simulink model "controllerComputedTorque"  (Simulink 8.0)
settings: Solver=FixedStepDiscrete  StartTime=0.0  StopTime=inf  FixedStep=1  RelTol=1e-3
InitFcn:
  | initSharedMem;
values from neighbouring files (symbols this model uses):
  k_pst = [ diag([k_pst_torso k_pst_arm k_pst_arm k_pst_leg k_pst_leg])    0*eye(25)   0*eye(25)]    [initCompleteForceControlSim.m]    (also in initPartialForceControl.m; initPartialForceControlSim.m)
  nj = 25    [initCompleteForceControlSim.m]    (also in initMonitor.m; initMonitorSim.m; initPartialForceControl.m; initPartialForceControlSim.m)
undefined symbols (not defined in the file or in its folder): DiscIntNeverNeededParam, k_com, k_pos
libraries: WBCLibrary x12, simulink x2, dspsigops x1
settings Model: Creator=daniele  LastModifiedBy=daniele
settings DebuggingCC: FcnCallInpInsideContextMsg=EnableAllAsWarning
settings GRTTargetCC: CombineOutputUpdateFcns=off  GRTInterface=on

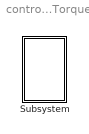
== system controllerComputedTorque ==
  Subsystem : Subsystem  mask{robotName='icub', Ts=0.01, localName='dynamicBalancing'}
      mask prompts: robotName "robot name"; localName "module name"

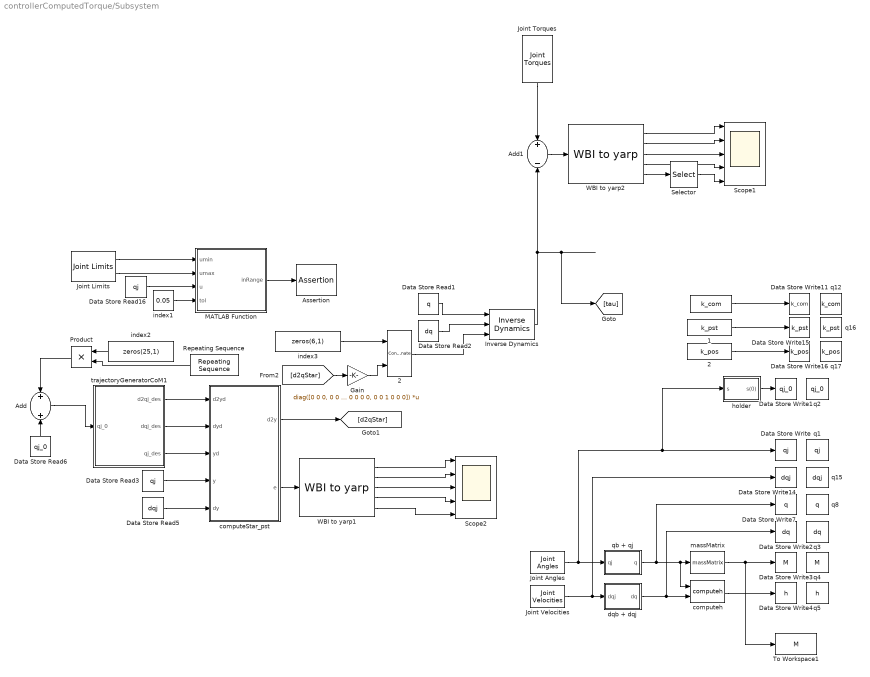
== system controllerComputedTorque/Subsystem ==
  "    " : Constant  Value=k_com
  "    1" : Constant  Value=k_pst
  "    2" : Constant  Value=k_pos
  " 2" : Concatenate  Mode=Multidimensional array
  Add : Sum  Inputs=+|+
  Add1 : Sum  Inputs=+|-
  Assertion : Assertion  Enabled=on
  Data Store Read1 : DataStoreRead  DataStoreName=q
  Data Store Read16 : DataStoreRead  DataStoreName=qj
  Data Store Read2 : DataStoreRead  DataStoreName=dq
  Data Store Read3 : DataStoreRead  DataStoreName=qj
  Data Store Read5 : DataStoreRead  DataStoreName=dqj
  Data Store Read6 : DataStoreRead  DataStoreName=qj_0
  Data Store Write : DataStoreWrite  Priority=-1  DataStoreName=qj
  Data Store Write1 : DataStoreWrite  Priority=-1  DataStoreName=qj_0
  Data Store Write11 : DataStoreWrite  Priority=-1  DataStoreName=k_com
  Data Store Write14 : DataStoreWrite  Priority=-1  DataStoreName=dqj
  Data Store Write15 : DataStoreWrite  Priority=-1  DataStoreName=k_pst
  Data Store Write16 : DataStoreWrite  Priority=-1  DataStoreName=k_pos
  Data Store Write2 : DataStoreWrite  Priority=-1  DataStoreName=dq
  Data Store Write3 : DataStoreWrite  Priority=-1  DataStoreName=M
  Data Store Write4 : DataStoreWrite  Priority=-1  DataStoreName=h
  Data Store Write7 : DataStoreWrite  Priority=-1  DataStoreName=q
  Gain : Gain  Gain=diag([0 0 0, 0 0 0 0 0, 0 0 0 0 0, 0 0 0 0 0 0, 0 0 1 0 0 0])  Multiplication=Matrix(K*u)
  Inverse Dynamics : WBCLibrary/wholeBodyModel/Dynamics/Inverse Dynamics  robotName=robotName  localName=localName
  Joint Angles : WBCLibrary/wholeBodyStates/Joint Angles  robotName=robotName  localName=localName
  Joint Limits : WBCLibrary/wholeBodyModel/Joint Limits  robotName=robotName  localName=localName
  Joint Torques : WBCLibrary/wholeBodyStates/Joint Torques  robotName=robotName  localName=localName
  Joint Velocities : WBCLibrary/wholeBodyStates/Joint Velocities  robotName=robotName  localName=localName
  MATLAB Function : MATLAB Function  TreatAsAtomicUnit=on
  Product : Product  RndMeth=Zero
  Repeating Sequence : simulink/Sources/Repeating Sequence  rep_seq_t=[0 1 2 3 4 ].*1000  rep_seq_y=[0 0 -0.1 -0.1 0]
  Scope1 : Scope  NumInputPorts=5
      settings: TimeRange=1400  YMin=-1~-0.5~-0.8~-0.2~-0.1  YMax=4~0.2~0.2~0.4~0.5
  Scope2 : Scope  NumInputPorts=5
      settings: TimeRange=1400  YMin=-0.5~-0.35~-0.6~-0.2~-0.75  YMax=3~0.1~0.1~0.3~0.75
  Selector : Selector  InputPortWidth=6  IndexOptions=Index vector (dialog)  Indices=[2 3]  OutputSizes=1
  To Workspace1 : ToWorkspace  VariableName=M  SampleTime=-1  SaveFormat=Structure
  WBI to yarp1 : WBCLibrary/Utilities/WBI to yarp
  WBI to yarp2 : WBCLibrary/Utilities/WBI to yarp
  computeStar_pst : Subsystem  mask{Kp=k_pst(1:25,1:25), Kd=k_pst(1:25,26:50), Ki=k_pst(1:25,51:75)}
  computeh : WBCLibrary/wholeBodyModel/Dynamics/computeh  val=7  robotname=robotName  localname=localName
  dqb + dqj : Subsystem
  holder : Subsystem
  index1 : Constant  Value=0.05  VectorParams1D=off
  index2 : Constant  Value=zeros(25,1)  VectorParams1D=off
  index3 : Constant  Value=zeros(6,1)  VectorParams1D=off
  massMatrix : WBCLibrary/wholeBodyModel/Dynamics/massMatrix  val=8  robotname=robotName  localname=localName
  q1 : DataStoreMemory  Priority=-1  DataStoreName=qj  ReadBeforeWriteMsg=warning  WriteAfterWriteMsg=warning  WriteAfterReadMsg=warning  InitialValue=zeros(nj,1)  VectorParams1D=off  OutDataTypeStr=double
  q12 : DataStoreMemory  Priority=-1  DataStoreName=k_com  ReadBeforeWriteMsg=warning  WriteAfterWriteMsg=warning  WriteAfterReadMsg=warning  InitialValue=k_com  VectorParams1D=off  OutDataTypeStr=double
  q15 : DataStoreMemory  Priority=-1  DataStoreName=dqj  ReadBeforeWriteMsg=warning  WriteAfterWriteMsg=warning  WriteAfterReadMsg=warning  InitialValue=zeros(nj,1)  VectorParams1D=off  OutDataTypeStr=double
  q16 : DataStoreMemory  Priority=-1  DataStoreName=k_pst  ReadBeforeWriteMsg=warning  WriteAfterWriteMsg=warning  WriteAfterReadMsg=warning  InitialValue=k_pst  VectorParams1D=off  OutDataTypeStr=double
  q17 : DataStoreMemory  Priority=-1  DataStoreName=k_pos  ReadBeforeWriteMsg=warning  WriteAfterWriteMsg=warning  WriteAfterReadMsg=warning  InitialValue=k_pos  VectorParams1D=off  OutDataTypeStr=double
  q2 : DataStoreMemory  Priority=-1  DataStoreName=qj_0  ReadBeforeWriteMsg=warning  WriteAfterWriteMsg=warning  WriteAfterReadMsg=warning  InitialValue=zeros(nj,1)  VectorParams1D=off  OutDataTypeStr=double
  q3 : DataStoreMemory  Priority=-1  DataStoreName=dq  ReadBeforeWriteMsg=warning  WriteAfterWriteMsg=warning  WriteAfterReadMsg=warning  InitialValue=zeros(nj+6,1)  VectorParams1D=off  OutDataTypeStr=double
  q4 : DataStoreMemory  Priority=-1  DataStoreName=M  ReadBeforeWriteMsg=warning  WriteAfterWriteMsg=warning  WriteAfterReadMsg=warning  InitialValue=zeros(nj+6,nj+6)  VectorParams1D=off  OutDataTypeStr=double
  q5 : DataStoreMemory  Priority=-1  DataStoreName=h  ReadBeforeWriteMsg=warning  WriteAfterWriteMsg=warning  WriteAfterReadMsg=warning  InitialValue=zeros(nj+6,1)  VectorParams1D=off  OutDataTypeStr=double
  q8 : DataStoreMemory  Priority=-1  DataStoreName=q  ReadBeforeWriteMsg=warning  WriteAfterWriteMsg=warning  WriteAfterReadMsg=warning  InitialValue=zeros(nj+16,1)  VectorParams1D=off  OutDataTypeStr=double
  qb + qj : Subsystem
  trajectoryGeneratorCoM1 : MATLAB Function  TreatAsAtomicUnit=on
  wires:
  qb + qj/1(q) -> massMatrix/1, computeh/1, Data Store Write7/1
  dqb + dqj/1(dq) -> computeh/2, Data Store Write2/1
  Joint Angles/1 -> qb + qj/1(qj), holder/1(s), Data Store Write/1
  holder/1(s(0)) -> Data Store Write1/1
  massMatrix/1 -> To Workspace1/1, Data Store Write3/1
  Joint Velocities/1 -> dqb + dqj/1(dqj), Data Store Write14/1
  "    "/1 -> Data Store Write11/1
  "    1"/1 -> Data Store Write15/1
  "    2"/1 -> Data Store Write16/1
  trajectoryGeneratorCoM1/1(d2qj_des) -> computeStar_pst/1(d2yd)
  trajectoryGeneratorCoM1/2(dqj_des) -> computeStar_pst/2(dyd)
  trajectoryGeneratorCoM1/3(qj_des) -> computeStar_pst/3(yd)
  Data Store Read3/1 -> computeStar_pst/4(y)
  Data Store Read5/1 -> computeStar_pst/5(dy)
  computeStar_pst/1(d2y) -> [d2qStar]
  Data Store Read1/1 -> Inverse Dynamics/1
  Data Store Read2/1 -> Inverse Dynamics/2
  index3/1 -> " 2"/1
  Inverse Dynamics/1 -> Add1/2, [tau]
  Data Store Read6/1 -> Add/2
  Add/1 -> trajectoryGeneratorCoM1/1(qj_0)
  Joint Limits/1 -> MATLAB Function/1(umin)
  Joint Limits/2 -> MATLAB Function/2(umax)
  Data Store Read16/1 -> MATLAB Function/3(u)
  index1/1 -> MATLAB Function/4(tol)
  MATLAB Function/1(inRange) -> Assertion/1
  Product/1 -> Add/1
  index2/1 -> Product/1
  Repeating Sequence/1 -> Product/2
  computeh/1 -> Data Store Write4/1
  WBI to yarp2/1 -> Scope1/1
  WBI to yarp2/2 -> Scope1/2
  WBI to yarp2/4 -> Scope1/4
  WBI to yarp2/5 -> Selector/1
  Joint Torques/1 -> Add1/1
  WBI to yarp2/3 -> Scope1/3
  Selector/1 -> Scope1/5
  WBI to yarp1/1 -> Scope2/1
  WBI to yarp1/2 -> Scope2/2
  WBI to yarp1/4 -> Scope2/4
  WBI to yarp1/3 -> Scope2/3
  WBI to yarp1/5 -> Scope2/5
  computeStar_pst/2(e) -> WBI to yarp1/1
  Add1/1 -> WBI to yarp2/1
  " 2"/1 -> Inverse Dynamics/3
  [d2qStar] -> Gain/1
  Gain/1 -> " 2"/2

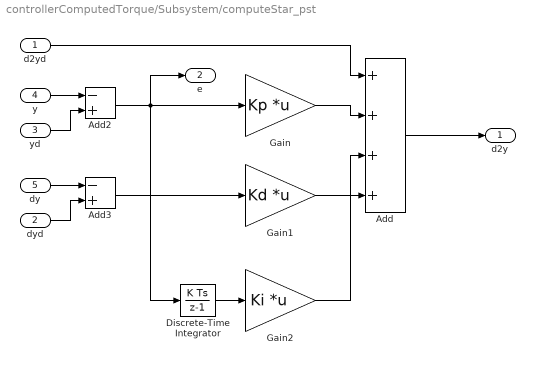
== system controllerComputedTorque/Subsystem/computeStar_pst ==
  d2yd : Inport
  dyd : Inport  Port=2
  yd : Inport  Port=3
  y : Inport  Port=4
  dy : Inport  Port=5
  Add : Sum  Inputs=++++
  Add2 : Sum  Inputs=-+
  Add3 : Sum  Inputs=-+
  Discrete-Time Integrator : DiscreteIntegrator  ICPrevOutput=DiscIntNeverNeededParam  ICPrevScaledInput=DiscIntNeverNeededParam
  Gain : Gain  Gain=Kp  Multiplication=Matrix(K*u)
  Gain1 : Gain  Gain=Kd  Multiplication=Matrix(K*u)
  Gain2 : Gain  Gain=Ki  Multiplication=Matrix(K*u)
  d2y : Outport
  e : Outport  Port=2
  wires:
  Discrete-Time Integrator/1 -> Gain2/1
  dyd/1 -> Add3/2
  yd/1 -> Add2/2
  d2yd/1 -> Add/1
  Add3/1 -> Gain1/1
  dy/1 -> Add3/1
  Add2/1 -> Discrete-Time Integrator/1, Gain/1, e/1
  y/1 -> Add2/1
  Add/1 -> d2y/1
  Gain2/1 -> Add/4
  Gain1/1 -> Add/3
  Gain/1 -> Add/2

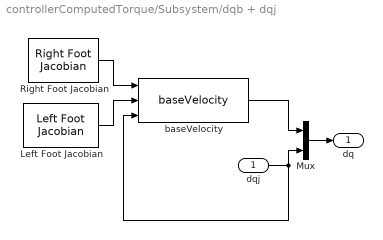
== system controllerComputedTorque/Subsystem/dqb + dqj ==
  dqj : Inport
  Left Foot Jacobian : WBCLibrary/wholeBodyModel/Jacobians/Left Foot Jacobian  robotName=robotName  localName=localName
  Mux : Mux  Inputs=2
  Right Foot Jacobian : WBCLibrary/wholeBodyModel/Jacobians/Right Foot Jacobian  robotName=robotName  localName=localName
  baseVelocity : WBCLibrary/Utilities/baseVelocity
  dq : Outport
  wires:
  Left Foot Jacobian/1 -> baseVelocity/2
  Right Foot Jacobian/1 -> baseVelocity/1
  baseVelocity/1 -> Mux/1
  dqj/1 -> baseVelocity/3, Mux/2
  Mux/1 -> dq/1

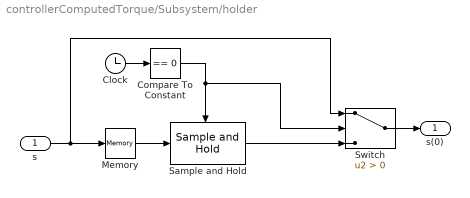
== system controllerComputedTorque/Subsystem/holder ==
  s : Inport
  Clock : Clock
  Compare To Constant : simulink/Logic and Bit Operations/Compare To Constant  relop===  const=0  OutDataTypeStr=boolean
  Memory : Memory
  Sample and Hold : dspsigops/Sample and Hold  trig=Falling edge  initCond=0  latchinput=off
  Switch : Switch  Criteria=u2 > Threshold
  s(0) : Outport
  wires:
  s/1 -> Switch/1, Memory/1
  Clock/1 -> Compare To Constant/1
  Compare To Constant/1 -> Sample and Hold/Trigger, Switch/2
  Sample and Hold/1 -> Switch/3
  Switch/1 -> s(0)/1
  Memory/1 -> Sample and Hold/1

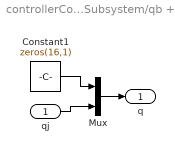
== system controllerComputedTorque/Subsystem/qb + qj ==
  qj : Inport
  Constant1 : Constant  Value=zeros(16,1)
  Mux : Mux  Inputs=2
  q : Outport
  wires:
  Mux/1 -> q/1
  Constant1/1 -> Mux/1
  qj/1 -> Mux/2

== matlab function Subsystem/MATLAB Function ==
  data: umin input double; umax input double; u input double; inRange output double; tol input double
function inRange = checkRange(umin, umax, u, tol)
%#codegen

res = u < umin + tol | u > umax - tol;
res = sum(res);
if res==0
    inRange = 1;
else
    inRange = 0;
    u < umin + tol | u > umax - tol
end

== matlab function Subsystem/trajectoryGeneratorCoM1 ==
  data: d2qj_des output double; dqj_des output double; qj_des output double; qj_0 input double
function [d2qj_des, dqj_des, qj_des]  = trajGen(qj_0)
%#codegen


qj_des    = qj_0;
dqj_des   = zeros(size(qj_0));
d2qj_des  = zeros(size(qj_0));
